simulink model "PubIfDecisionTOS_MDL"  (R2020b)
settings: configuration reference "DspaceConfig" (kept outside this file)
PostLoadFcn:
  | if any(exist('dsrtsu_mdlpostloadfcn', 'file') ~= 0), dsrtsu_mdlpostloadfcn('Execute', bdroot); end
InitFcn:
  | , if any(exist('dsmpb_private', 'file') ~= 0), dsmpb_private('dsmpb_mdlclblib', 'Init', bdroot); end,
undefined symbols (not defined in the file or in its folder): C_TOS_ACCEgoRAxletoFbumplength_m, C_TOS_ACCTargetFront_Flag, C_TOS_AEBJAPedObjDxThre_Val, C_TOS_AEBJAPedObjDyThre_Val, C_TOS_AEBJATargetSize_Val, C_TOS_AEBJAVehObjDxThre_Val, C_TOS_AEBJAVehObjDyThre_Val, C_TOS_AEBJuncPedTargetSize_Val, C_TOS_AEBLatObjDxThre_Val, C_TOS_AEBLatPedDyThre_Val, C_TOS_AEBLatTargetSize_Val, C_TOS_AEBLongTargetInEgoFront_Flag, C_TOS_axAbsGround_Parameter, C_TOS_CameraConfirmedFlag, C_TOS_CNsubjWidth, C_TOS_CurrentLaneCoreMinWidth_Val, C_TOS_CutInProb_Val_Zero, C_TOS_CutOutProb_Val_Zero, C_TOS_D2R_Val, C_TOS_DefaultValueObjectToCenterLine_dy, C_TOS_EgoCarWidth_Val, C_TOS_EgoDxRefPoint_m, C_TOS_EgoRAxletoFbumplength_m, C_TOS_HalfWidthVehicle_Con, C_TOS_HWA_CurrentLaneFlag, C_TOS_HWA_LeftLaneFlag, C_TOS_HWA_MovingDir_Vaild, C_TOS_HWA_MovState_Vaild, C_TOS_HWA_RightLaneFlag, C_TOS_LaneLineCourseErrorFront, C_TOS_LaneLineCourseErrorRear, C_TOS_MotorbikeDefaultWidth_m, C_TOS_NumberOfEffectiveTargets, C_TOS_Obj_Age_Val, C_TOS_Objdx_Constraint_Val, C_TOS_ObjectDefaultWidth_m, C_TOS_ObjInCurrentLane_Val, C_TOS_ObjInCurrentLaneValid, C_TOS_ObjInLeftLaneValid, C_TOS_ObjInRightLaneValid, C_TOS_ObjNotInCurrentLane_Val, C_TOS_ObjNotREElementType, C_TOS_ObjPredictDis_dy_ConstantVal_Zeros, C_TOS_ObjToCenterLine_ConstantVal_Zeros, C_TOS_OFMObjIDInvilad_Val, C_TOS_PIL_LatDisCons_Val_zero, C_TOS_PIL_ObjectCutInFlag_b, C_TOS_PIL_ObjectCutOutFlag_b, C_TOS_PIL_ObjLaneProb_al_Val, C_TOS_PP_ObjFusType_FC_Confirm_b, C_TOS_PP_ObjFusType_FC_FR_Confirm_b, C_TOS_PP_ObjFusType_FR_Confirm_b, C_TOS_RE_80BoolDefault_Val, C_TOS_RE_80Single181Default_Val, C_TOS_RE_80Single255Default_Val, C_TOS_RE_80Uint8Default_Val, C_TOS_RE_D2R, C_TOS_RE_D_180_Val, C_TOS_RE_InvalidObjectID_Val, C_TOS_RE_InvalidTargetChainDir_Val ... (+142)
libraries: simulink x1650, TOS_LIB x361, canfdmsglib x14
(part 19 of 69)

== system PubIfDecisionTOS_MDL/TOS_20201112/TOS_2012080320/TOS/ACC/TOS_ACCCurrentLane/ACC_CurrentLane_Target/TOS_ACC_P1 ==
  ACC_P0_P1_Index : Inport
  Object_ID : Inport  Port=2
  Object_Fus_Type : Inport  Port=3
  object_MovingState : Inport  Port=4
  PP_ObjMovingDirSignalProcessing : Inport  Port=5
  Object_HeadingAngle : Inport  Port=6
  Object_DX : Inport  Port=7
  TOS_TLJ_SameLaneConfirm_Flag : Inport  Port=8
  Object_Type : Inport  Port=9
  Object_ObstacleProb : Inport  Port=10
  Object_DY : Inport  Port=11
  PP_ObjFusType_FC_FR_Confirm : Inport  Port=12
  PP_ObjFusType_FR_Confirm : Inport  Port=13
  PP_ObjFusType_FC_Confirm : Inport  Port=14
  Object_VX : Inport  Port=15
  Object_VY : Inport  Port=16
  VIE_EgoVelocity : Inport  Port=17
  SteerWheelAng : Inport  Port=18
  PIL_OverlapRatio : Inport  Port=19
  ACC_TargetP1_ID_K1 : Inport  Port=20
  ACC_TargetP1_ID_K2 : Inport  Port=21
  ACC_TargetP1_MovState_K1 : Inport  Port=22
  ACC_TargetP1_MovState_K2 : Inport  Port=23
  LM_LR_Line04_dDisStart : Inport  Port=24
  LM_LR_Line04_dDisEnd : Inport  Port=25
  LM_LR_Line05_dDisStart : Inport  Port=26
  LM_LR_Line05_dDisEnd : Inport  Port=27
  LM_LR_Line06_dDisStart : Inport  Port=28
  LM_LR_Line06_dDisEnd : Inport  Port=29
  LM_LR_Line04_pC2 : Inport  Port=30
  LM_LR_Line05_pC2 : Inport  Port=31
  LM_LR_Line06_pC2 : Inport  Port=32
  LM_LR_Line04_fCamValid : Inport  Port=33
  LM_LR_Line05_fCamValid : Inport  Port=34
  LM_LR_Line06_fCamValid : Inport  Port=35
  LM_LR_Line04_pC0 : Inport  Port=36
  LM_RL_Line04_pC0 : Inport  Port=37
  ACC_P1_Targe : Subsystem
  ACC_P1_TargeDefault : Subsystem  TreatAsAtomicUnit=on
  Compare To Constant : simulink/Logic and Bit Operations/Compare To Constant  relop===  const=C_TOS_OFMObjIDInvilad_Val  OutDataTypeStr=boolean
      settings: AttributesFormatString=C_TOS_OFMObjIDInvilad_Val = 0
  Constant1 : Constant  Value=0  OutDataTypeStr=uint8
  If : If  IfExpression=u1 ~= 0
  Merge{,1..18} (19 alike) : Merge
  Selector17 : Selector  InputPortWidth=2  IndexOptions=Index vector (dialog)  Indices=2  OutputSizes=1
  Switch1 : Switch  Criteria=u2 ~= 0
  TOS_ACC_P1_Index : Outport
  TOS_ACC_FusionType_ObserVale : Outport  Port=2
  TOS_ACC_TrgMovDir_ObserVale : Outport  Port=3
  TOS_ACC_TargetDxConfirm_ObserVale : Outport  Port=4
  TOS_ACC_ObjType_ObserVale : Outport  Port=5
  TOS_ACC_ObstacleProb_ObserVale : Outport  Port=6
  TOS_ACC_DyConfirm_ObserVale : Outport  Port=7
  TOS_ACC_TrgMovDirFlag_1_ObserVale : Outport  Port=8
  TOS_ACC_TrgMovDirFlag_2_ObserVale : Outport  Port=9
  TOS_ACC_TrgMovDirFlag_3_ObserVale : Outport  Port=10
  TOS_ACC_TrgMovDirFlag_4_ObserVale : Outport  Port=11
  TOS_ACC_TrgMovDirFlag_5_ObserVale : Outport  Port=12
  TOS_ACC_TrgMovDirFlag_6_ObserVale : Outport  Port=13
  TOS_ACC_DyConfirm_1_ObserVale : Outport  Port=14
  TOS_ACC_DyConfirm_2_ObserVale : Outport  Port=15
  TOS_ACC_DyConfirm_3_ObserVale : Outport  Port=16
  TOS_ACC_DyConfirm_4_OverlapRatio_ObserVale : Outport  Port=17
  TOS_ACC_DyConfirm_5_OverlapConfirm_ObserVale : Outport  Port=18
  TOS_ACC_DyConfirm_ALL_6_ObserVale : Outport  Port=19
  wires:
  LM_RL_Line04_pC0/1 -> ACC_P1_Targe/37(LM_RL_Line04_pC0)  "LM_RL_Line04_pC0"
  LM_LR_Line04_pC0/1 -> ACC_P1_Targe/36(LM_LR_Line04_pC0)  "LM_LR_Line04_pC0"
  ACC_P1_TargeDefault/19(TOS_ACC_DyConfirm_ALL_6_ObserVale1) -> Merge18/1
  Merge18/1 -> TOS_ACC_DyConfirm_ALL_6_ObserVale/1
  ACC_P1_Targe/19(TOS_ACC_DyConfirm_ALL_6_ObserVale) -> Merge18/2
  ACC_P1_TargeDefault/18(TOS_ACC_DyConfirm_5_OverlapConfirm_ObserVale) -> Merge17/1
  ACC_P1_TargeDefault/17(TOS_ACC_DyConfirm_4_OverlapRatio_ObserVale) -> Merge15/1
  ACC_P1_TargeDefault/16(TOS_ACC_DyConfirm_3_ObserVale) -> Merge14/1
  ACC_P1_TargeDefault/15(TOS_ACC_DyConfirm_2_ObserVale) -> Merge13/1
  ACC_P1_TargeDefault/14(TOS_ACC_DyConfirm_1_ObserVale) -> Merge16/1
  ACC_P1_TargeDefault/13(TOS_ACC_TrgMovDirFlag_6_ObserVale) -> Merge8/1
  ACC_P1_TargeDefault/12(TOS_ACC_TrgMovDirFlag_5_ObserVale) -> Merge12/1
  ACC_P1_TargeDefault/11(TOS_ACC_TrgMovDirFlag_4_ObserVale) -> Merge11/1
  ACC_P1_TargeDefault/10(TOS_ACC_TrgMovDirFlag_3_ObserVale) -> Merge10/1
  ACC_P1_TargeDefault/9(TOS_ACC_TrgMovDirFlag_2_ObserVale) -> Merge9/1
  ACC_P1_TargeDefault/8(TOS_ACC_TrgMovDirFlag_1_ObserVale) -> Merge7/1
  ACC_P1_TargeDefault/7(TOS_ACC_DyConfirm_ObserVale) -> Merge6/1
  ACC_P1_TargeDefault/6(TOS_ACC_ObstacleProb_ObserVale) -> Merge5/1
  ACC_P1_TargeDefault/5(TOS_ACC_ObjType_ObserVale) -> Merge4/1
  ACC_P1_TargeDefault/4(TOS_ACC_TargetDxConfirm_ObserVale) -> Merge3/1
  ACC_P1_TargeDefault/3(TOS_ACC_TrgMovDir_ObserVale) -> Merge2/1
  ACC_P1_TargeDefault/2(TOS_ACC_FusionType_ObserVale) -> Merge1/1
  ACC_P1_TargeDefault/1(ACC_P1_TargeConfirm) -> Merge/1
  ACC_P1_Targe/18(TOS_ACC_DyConfirm_5_OverlapConfirm_ObserVale) -> Merge17/2
  Merge17/1 -> TOS_ACC_DyConfirm_5_OverlapConfirm_ObserVale/1
  LM_LR_Line06_fCamValid/1 -> ACC_P1_Targe/35(LM_LR_Line06_fCamValid)
  LM_LR_Line05_fCamValid/1 -> ACC_P1_Targe/34(LM_LR_Line05_fCamValid)
  LM_LR_Line04_fCamValid/1 -> ACC_P1_Targe/33(LM_LR_Line04_fCamValid)
  LM_LR_Line06_pC2/1 -> ACC_P1_Targe/32(LM_LR_Line06_pC2)
  LM_LR_Line05_pC2/1 -> ACC_P1_Targe/31(LM_LR_Line05_pC2)
  LM_LR_Line04_pC2/1 -> ACC_P1_Targe/30(LM_LR_Line04_pC2)
  LM_LR_Line06_dDisEnd/1 -> ACC_P1_Targe/29(LM_LR_Line06_dDisEnd)
  LM_LR_Line06_dDisStart/1 -> ACC_P1_Targe/28(LM_LR_Line06_dDisStart)
  LM_LR_Line05_dDisEnd/1 -> ACC_P1_Targe/27(LM_LR_Line05_dDisEnd)
  LM_LR_Line05_dDisStart/1 -> ACC_P1_Targe/26(LM_LR_Line05_dDisStart)
  LM_LR_Line04_dDisEnd/1 -> ACC_P1_Targe/25(LM_LR_Line04_dDisEnd)
  LM_LR_Line04_dDisStart/1 -> ACC_P1_Targe/24(LM_LR_Line04_dDisStart)
  ACC_P1_Targe/14(TOS_ACC_DyConfirm_1_ObserVale) -> Merge16/2
  Merge16/1 -> TOS_ACC_DyConfirm_1_ObserVale/1
  Switch1/1 -> TOS_ACC_P1_Index/1
  Selector17/1 -> Compare To Constant/1, [ACC_P1_Index]
  Merge15/1 -> TOS_ACC_DyConfirm_4_OverlapRatio_ObserVale/1
  Merge14/1 -> TOS_ACC_DyConfirm_3_ObserVale/1
  Merge13/1 -> TOS_ACC_DyConfirm_2_ObserVale/1
  ACC_P1_Targe/17(TOS_ACC_DyConfirm_4_OverlapRatio_ObserVale) -> Merge15/2
  ACC_P1_Targe/16(TOS_ACC_DyConfirm_3_ObserVale) -> Merge14/2
  ACC_P1_Targe/15(TOS_ACC_DyConfirm_2_ObserVale) -> Merge13/2
  ACC_P1_Targe/12(TOS_ACC_TrgMovDirFlag_5_ObserVale) -> Merge12/2
  ACC_P1_Targe/11(TOS_ACC_TrgMovDirFlag_4_ObserVale) -> Merge11/2
  ACC_P1_Targe/10(TOS_ACC_TrgMovDirFlag_3_ObserVale) -> Merge10/2
  ACC_P1_Targe/9(TOS_ACC_TrgMovDirFlag_2_ObserVale) -> Merge9/2
  Merge12/1 -> TOS_ACC_TrgMovDirFlag_5_ObserVale/1
  Merge11/1 -> TOS_ACC_TrgMovDirFlag_4_ObserVale/1
  Merge10/1 -> TOS_ACC_TrgMovDirFlag_3_ObserVale/1
  Merge9/1 -> TOS_ACC_TrgMovDirFlag_2_ObserVale/1
  Merge8/1 -> TOS_ACC_TrgMovDirFlag_6_ObserVale/1
  ACC_P1_Targe/13(TOS_ACC_TrgMovDirFlag_6_ObserVale) -> Merge8/2
  Object_ID/1 -> ACC_P1_Targe/23(ObjectID)
  ACC_TargetP1_MovState_K2/1 -> ACC_P1_Targe/22(ACC_Target_MovState_K2)
  ACC_TargetP1_MovState_K1/1 -> ACC_P1_Targe/21(ACC_Target_MovState_K1)
  ACC_TargetP1_ID_K2/1 -> ACC_P1_Targe/20(ACC_Target_ID_K2)
  ACC_TargetP1_ID_K1/1 -> ACC_P1_Targe/19(ACC_Target_ID_K1)
  Merge7/1 -> TOS_ACC_TrgMovDirFlag_1_ObserVale/1
  ACC_P1_Targe/8(TOS_ACC_TrgMovDirFlag_1_ObserVale) -> Merge7/2
  PIL_OverlapRatio/1 -> ACC_P1_Targe/18(PIL_OverlapRatio)
  SteerWheelAng/1 -> ACC_P1_Targe/17(SteerWheelAng)
  VIE_EgoVelocity/1 -> ACC_P1_Targe/16(VIE_EgoVelocity)
  Object_VX/1 -> ACC_P1_Targe/14(Object_VX)
  Object_VY/1 -> ACC_P1_Targe/15(Object_VY)
  PP_ObjFusType_FR_Confirm/1 -> ACC_P1_Targe/12(PP_ObjFusType_FR_Confirm)
  PP_ObjFusType_FC_FR_Confirm/1 -> ACC_P1_Targe/11(PP_ObjFusType_FC_FR_Confirm)
  PP_ObjFusType_FC_Confirm/1 -> ACC_P1_Targe/13(PP_ObjFusType_FC_Confirm)
  If/2 -> ACC_P1_Targe/Action
  ACC_P1_Targe/7(TOS_ACC_DyConfirm_ObserVale) -> Merge6/2
  ACC_P1_Targe/6(TOS_ACC_ObstacleProb_ObserVale) -> Merge5/2
  ACC_P1_Targe/5(TOS_ACC_ObjType_ObserVale) -> Merge4/2
  ACC_P1_Targe/4(TOS_ACC_TargetDxConfirm_ObserVale) -> Merge3/2
  ACC_P1_Targe/3(TOS_ACC_TrgMovDir_ObserVale) -> Merge2/2
  ACC_P1_Targe/2(TOS_ACC_FusionType_ObserVale) -> Merge1/2
  ACC_P1_Targe/1(ACC_P1_TargeConfirm) -> Merge/2
  Object_DY/1 -> ACC_P1_Targe/10(Object_DY)
  Object_ObstacleProb/1 -> ACC_P1_Targe/9(Object_ObstacleProb)
  Object_Type/1 -> ACC_P1_Targe/8(Object_Type)
  TOS_TLJ_SameLaneConfirm_Flag/1 -> ACC_P1_Targe/7(TOS_TLJ_SameLaneConfirm_Flag)
  Object_DX/1 -> ACC_P1_Targe/6(Object_DX)
  Object_HeadingAngle/1 -> ACC_P1_Targe/5(Object_HeadingAngle)
  PP_ObjMovingDirSignalProcessing/1 -> ACC_P1_Targe/4(PP_ObjMovingDirSignalProcessing)
  object_MovingState/1 -> ACC_P1_Targe/3(object_MovingState)
  Object_Fus_Type/1 -> ACC_P1_Targe/2(Object_Fus_Type)
  [ACC_P1_Index] -> ACC_P1_Targe/1(ACC_P1_Index)
  ACC_P0_P1_Index/1 -> Selector17/1
  Constant1/1 -> Switch1/3
  Merge/1 -> Switch1/2
  [ACC_P1_Index] -> Switch1/1
  Merge6/1 -> TOS_ACC_DyConfirm_ObserVale/1
  Merge5/1 -> TOS_ACC_ObstacleProb_ObserVale/1
  Merge4/1 -> TOS_ACC_ObjType_ObserVale/1
  Merge3/1 -> TOS_ACC_TargetDxConfirm_ObserVale/1
  Merge2/1 -> TOS_ACC_TrgMovDir_ObserVale/1
  Merge1/1 -> TOS_ACC_FusionType_ObserVale/1
  Compare To Constant/1 -> If/1
  If/1 -> ACC_P1_TargeDefault/Action

== system PubIfDecisionTOS_MDL/TOS_20201112/TOS_2012080320/TOS/ACC/TOS_ACCCurrentLane/ACC_Object_PreConfirm/ACC_P0_P1_Object_TargPreConfirm ==
  PP_ObjFusType_FC_FR_Confirm : Inport  Partition=on  PartitionDimension=1  PartitionWidth=1  PartitionOffset=0
  PP_ObjFusType_FR_Confirm : Inport  Port=2  Partition=on  PartitionDimension=1  PartitionWidth=1  PartitionOffset=0
  PP_ObjFusType_FC_Confirm : Inport  Port=3  Partition=on  PartitionDimension=1  PartitionWidth=1  PartitionOffset=0
  Object_ID : Inport  Port=4  OutDataTypeStr=uint8  Partition=on  PartitionDimension=1  PartitionWidth=1  PartitionOffset=0
  Obj_MovingState : Inport  Port=5  Partition=on  PartitionDimension=1  PartitionWidth=1  PartitionOffset=0
  Obj_Dx : Inport  Port=6  Partition=on  PartitionDimension=1  PartitionWidth=1  PartitionOffset=0
  Object_ObstacleProb : Inport  Port=7  Partition=on  PartitionDimension=1  PartitionWidth=1  PartitionOffset=0
  Object_DY : Inport  Port=8  Partition=on  PartitionDimension=1  PartitionWidth=1  PartitionOffset=0
  Object_ObjType : Inport  Port=9  Partition=on  PartitionDimension=1  PartitionWidth=1  PartitionOffset=0
  TOS_TLJ_SameLaneConfirm_Flag : Inport  Port=10  Partition=on  PartitionDimension=1  PartitionWidth=1  PartitionOffset=0
  LM_LR_Line04_fCamValid : Inport  Port=11
  LM_LR_Line05_fCamValid : Inport  Port=12
  LM_LR_Line06_fCamValid : Inport  Port=13
  ACC_TargetP0_ID_K1 : Inport  Port=14
  ACC_TargetP0_Dx_K1 : Inport  Port=15
  PIL_OverlapRatio : Inport  Port=16  Partition=on  PartitionDimension=1  PartitionWidth=1  PartitionOffset=0
  PIL_OverlapRatio_K1 : Inport  Port=17  Partition=on  PartitionDimension=1  PartitionWidth=1  PartitionOffset=0
  PIL_OverlapRatio_K2 : Inport  Port=18  Partition=on  PartitionDimension=1  PartitionWidth=1  PartitionOffset=0
  LM_LR_Line04_dDisStart : Inport  Port=19
  LM_LR_Line04_dDisEnd : Inport  Port=20
  LM_LR_Line05_dDisStart : Inport  Port=21
  LM_LR_Line05_dDisEnd : Inport  Port=22
  LM_LR_Line06_dDisStart : Inport  Port=23
  LM_LR_Line06_dDisEnd : Inport  Port=24
  PP_REElementType : Inport  Port=25  Partition=on  PartitionDimension=1  PartitionWidth=1  PartitionOffset=0
  ACC_P0_P1_Object_TargPreConfirm : Subsystem
  ACC_P0_P1_Object_TargPreConfirmDefault : Subsystem  TreatAsAtomicUnit=on
  Compare To Constant : simulink/Logic and Bit Operations/Compare To Constant  relop===  const=C_TOS_OFMObjIDInvilad_Val  OutDataTypeStr=boolean
      settings: AttributesFormatString=C_TOS_OFMObjIDInvilad_Val = 0
  For Each : ForEach  DisableCoverage=on
  If : If  IfExpression=u1 ~= 0
  Merge{,1..10} (11 alike) : Merge
  TOS_ACC_P0_P1_TargetPre_1_ConditionFlag_ObserVale : Outport  ConcatenationDimension=1
  TOS_ACC_P0_P1_TargetPre_2_OverlapThre_ObserVale : Outport  Port=2  ConcatenationDimension=1
  TOS_ACC_P0_P1_TargetPre_3_SameLane_Flag_ObserVale : Outport  Port=3  ConcatenationDimension=1
  TOS_ACC_P0_P1_TargetPre_SameLaneFlag : Outport  Port=4  ConcatenationDimension=1
  TOS_ACC_P0_P1_TargetPre_FiltFlag : Outport  Port=5  ConcatenationDimension=1
  TOS_ACC_P0_P1_TargetPre_FusionTypeFlag_ObserVale : Outport  Port=6  ConcatenationDimension=1
  TOS_ACC_P0_P1_TargetPre_PassedbyTarget_Flag_ObserVale : Outport  Port=7  ConcatenationDimension=1
  TOS_ACC_P0_P1_TargetPre_FenceFlag_ObserVale : Outport  Port=8  ConcatenationDimension=1
  TOS_ACC_P0_P1_TargetPre_ObjType_ObserVale : Outport  Port=9  ConcatenationDimension=1
  TOS_ACC_P0_P1_TargetPre_OverlapThre_Val_ObserVale : Outport  Port=10  ConcatenationDimension=1
  TOS_ACC_P0_P1_TargetPre_REElementType_ObserVale : Outport  Port=11  ConcatenationDimension=1
  wires:
  PP_ObjFusType_FC_FR_Confirm/1 -> ACC_P0_P1_Object_TargPreConfirm/2(PP_ObjFusType_FC_FR_Confirm)
  PP_ObjFusType_FR_Confirm/1 -> ACC_P0_P1_Object_TargPreConfirm/3(PP_ObjFusType_FR_Confirm)
  Compare To Constant/1 -> If/1
  Object_ID/1 -> [Object_ID], Compare To Constant/1
  If/1 -> ACC_P0_P1_Object_TargPreConfirmDefault/Action
  If/2 -> ACC_P0_P1_Object_TargPreConfirm/Action
  PP_ObjFusType_FC_Confirm/1 -> ACC_P0_P1_Object_TargPreConfirm/4(PP_ObjFusType_FC_Confirm)
  Obj_MovingState/1 -> ACC_P0_P1_Object_TargPreConfirm/5(Obj_MovingState)
  Obj_Dx/1 -> ACC_P0_P1_Object_TargPreConfirm/6(Obj_Dx)
  Object_ObstacleProb/1 -> ACC_P0_P1_Object_TargPreConfirm/7(Object_ObstacleProb)
  Object_DY/1 -> ACC_P0_P1_Object_TargPreConfirm/8(Object_DY)
  ACC_TargetP0_ID_K1/1 -> ACC_P0_P1_Object_TargPreConfirm/14(ACC_TargetP0_ID_K1)
  ACC_TargetP0_Dx_K1/1 -> ACC_P0_P1_Object_TargPreConfirm/15(ACC_TargetP0_Dx_K1)
  [Object_ID] -> ACC_P0_P1_Object_TargPreConfirm/1(Object_ID)
  Object_ObjType/1 -> ACC_P0_P1_Object_TargPreConfirm/9(Object_ObjType)
  PIL_OverlapRatio/1 -> ACC_P0_P1_Object_TargPreConfirm/16(PIL_OverlapRatio)
  TOS_TLJ_SameLaneConfirm_Flag/1 -> ACC_P0_P1_Object_TargPreConfirm/10(TOS_TLJ_SameLaneConfirm_Flag)
  Merge/1 -> TOS_ACC_P0_P1_TargetPre_1_ConditionFlag_ObserVale/1
  Merge1/1 -> TOS_ACC_P0_P1_TargetPre_2_OverlapThre_ObserVale/1
  Merge2/1 -> TOS_ACC_P0_P1_TargetPre_3_SameLane_Flag_ObserVale/1
  Merge3/1 -> TOS_ACC_P0_P1_TargetPre_SameLaneFlag/1
  Merge4/1 -> TOS_ACC_P0_P1_TargetPre_FiltFlag/1
  Merge5/1 -> TOS_ACC_P0_P1_TargetPre_FusionTypeFlag_ObserVale/1
  Merge6/1 -> TOS_ACC_P0_P1_TargetPre_PassedbyTarget_Flag_ObserVale/1
  Merge7/1 -> TOS_ACC_P0_P1_TargetPre_ObjType_ObserVale/1
  Merge8/1 -> TOS_ACC_P0_P1_TargetPre_OverlapThre_Val_ObserVale/1
  ACC_P0_P1_Object_TargPreConfirm/1(TOS_ACC_P0_P1_TargetPre_1_ConditionFlag_ObserVale) -> Merge/2
  ACC_P0_P1_Object_TargPreConfirm/10(TOS_ACC_P0_P1_TargetPre_OverlapThre_Val_ObserVale) -> Merge8/2
  ACC_P0_P1_Object_TargPreConfirm/2(TOS_ACC_P0_P1_TargetPre_2_OverlapThre_ObserVale) -> Merge1/2
  ACC_P0_P1_Object_TargPreConfirm/3(TOS_ACC_P0_P1_TargetPre_3_SameLane_Flag_ObserVale) -> Merge2/2
  ACC_P0_P1_Object_TargPreConfirm/4(TOS_ACC_P0_P1_TargetPre_SameLaneFlag) -> Merge3/2
  ACC_P0_P1_Object_TargPreConfirm/5(TOS_ACC_P0_P1_TargetPre_FiltFlag) -> Merge4/2
  ACC_P0_P1_Object_TargPreConfirm/6(TOS_ACC_P0_P1_TargetPre_FusionTypeFlag_ObserVale) -> Merge5/2
  ACC_P0_P1_Object_TargPreConfirm/7(TOS_ACC_P0_P1_TargetPre_PassedbyTarget_Flag_ObserVale) -> Merge6/2
  ACC_P0_P1_Object_TargPreConfirm/8(TOS_ACC_P0_P1_TargetPre_FenceFlag_ObserVale) -> Merge9/2
  ACC_P0_P1_Object_TargPreConfirm/9(TOS_ACC_P0_P1_TargetPre_ObjType_ObserVale) -> Merge7/2
  ACC_P0_P1_Object_TargPreConfirmDefault/1(TOS_ACC_P0_P1_TargetPre_1_ConditionFlag_ObserVale) -> Merge/1
  ACC_P0_P1_Object_TargPreConfirmDefault/2(TOS_ACC_P0_P1_TargetPre_2_OverlapThre_ObserVale) -> Merge1/1
  ACC_P0_P1_Object_TargPreConfirmDefault/3(TOS_ACC_P0_P1_TargetPre_3_SameLane_Flag_ObserVale) -> Merge2/1
  ACC_P0_P1_Object_TargPreConfirmDefault/4(TOS_ACC_P0_P1_TargetPre_SameLaneFlag) -> Merge3/1
  ACC_P0_P1_Object_TargPreConfirmDefault/5(TOS_ACC_P0_P1_TargetPre_FiltFlag) -> Merge4/1
  ACC_P0_P1_Object_TargPreConfirmDefault/6(TOS_ACC_P0_P1_TargetPre_FusionTypeFlag_ObserVale) -> Merge5/1
  ACC_P0_P1_Object_TargPreConfirmDefault/7(TOS_ACC_P0_P1_TargetPre_PassedbyTarget_Flag_ObserVale) -> Merge6/1
  ACC_P0_P1_Object_TargPreConfirmDefault/8(TOS_ACC_P0_P1_TargetPre_FenceFlag_ObserVale) -> Merge9/1
  ACC_P0_P1_Object_TargPreConfirmDefault/9(TOS_ACC_P0_P1_TargetPre_ObjType_ObserVale) -> Merge7/1
  ACC_P0_P1_Object_TargPreConfirmDefault/10(TOS_ACC_P0_P1_TargetPre_OverlapThre_Val_ObserVale) -> Merge8/1
  Merge9/1 -> TOS_ACC_P0_P1_TargetPre_FenceFlag_ObserVale/1
  PIL_OverlapRatio_K1/1 -> ACC_P0_P1_Object_TargPreConfirm/17(PIL_OverlapRatio_K1)
  PIL_OverlapRatio_K2/1 -> ACC_P0_P1_Object_TargPreConfirm/18(PIL_OverlapRatio_K2)
  LM_LR_Line04_fCamValid/1 -> ACC_P0_P1_Object_TargPreConfirm/11(LM_LR_Line04_fCamValid)
  LM_LR_Line05_fCamValid/1 -> ACC_P0_P1_Object_TargPreConfirm/12(LM_LR_Line05_fCamValid)
  LM_LR_Line06_fCamValid/1 -> ACC_P0_P1_Object_TargPreConfirm/13(LM_LR_Line06_fCamValid)
  LM_LR_Line04_dDisStart/1 -> ACC_P0_P1_Object_TargPreConfirm/19(LM_LR_Line04_dDisStart)
  LM_LR_Line04_dDisEnd/1 -> ACC_P0_P1_Object_TargPreConfirm/20(LM_LR_Line04_dDisEnd)
  LM_LR_Line05_dDisStart/1 -> ACC_P0_P1_Object_TargPreConfirm/21(LM_LR_Line05_dDisStart)
  LM_LR_Line05_dDisEnd/1 -> ACC_P0_P1_Object_TargPreConfirm/22(LM_LR_Line05_dDisEnd)
  LM_LR_Line06_dDisStart/1 -> ACC_P0_P1_Object_TargPreConfirm/23(LM_LR_Line06_dDisStart)
  LM_LR_Line06_dDisEnd/1 -> ACC_P0_P1_Object_TargPreConfirm/24(LM_LR_Line06_dDisEnd)
  PP_REElementType/1 -> ACC_P0_P1_Object_TargPreConfirm/25(PP_REElementType)
  Merge10/1 -> TOS_ACC_P0_P1_TargetPre_REElementType_ObserVale/1
  ACC_P0_P1_Object_TargPreConfirm/11(TOS_ACC_P0_P1_TargetPre_REElementType_ObserVale) -> Merge10/2
  ACC_P0_P1_Object_TargPreConfirmDefault/11(TOS_ACC_P0_P1_TargetPre_REElementType_ObserVale) -> Merge10/1

== system PubIfDecisionTOS_MDL/TOS_20201112/TOS_2012080320/TOS/ACC/TOS_ACCLeftLane/ACC_LeftLane_Target/TOS_ACC_P2 ==
  TOS_ACC_P2_P4_Index : Inport
  Object_ID : Inport  Port=2
  Object_Fus_Type : Inport  Port=3
  object_MovingState : Inport  Port=4
  PP_ObjMovingDirSignalProcessing : Inport  Port=5
  Object_HeadingAngle : Inport  Port=6
  Object_DX : Inport  Port=7
  Object_Type : Inport  Port=8
  Object_ObstacleProb : Inport  Port=9
  Object_DY : Inport  Port=10
  PP_ObjFusType_FC_FR_Confirm : Inport  Port=11
  PP_ObjFusType_FR_Confirm : Inport  Port=12
  PP_ObjFusType_FC_Confirm : Inport  Port=13
  Object_VX : Inport  Port=14
  Object_VY : Inport  Port=15
  VIE_EgoVelocity : Inport  Port=16
  SteerWheelAng : Inport  Port=17
  ACC_TargetP2_ID_K1 : Inport  Port=18
  ACC_TargetP2_ID_K2 : Inport  Port=19
  ACC_TargetP2_MovState_K1 : Inport  Port=20
  ACC_TargetP2_MovState_K2 : Inport  Port=21
  ACC_P2_Targe : Subsystem
  ACC_P2_TargeDefault : Subsystem  TreatAsAtomicUnit=on
  Compare To Constant : simulink/Logic and Bit Operations/Compare To Constant  relop===  const=C_TOS_OFMObjIDInvilad_Val  OutDataTypeStr=boolean
      settings: AttributesFormatString=C_TOS_OFMObjIDInvilad_Val = 0
  Constant1 : Constant  Value=0  OutDataTypeStr=uint8
  If : If  IfExpression=u1 ~= 0
  Merge{,1..5,7..12} (12 alike) : Merge
  Selector17 : Selector  InputPortWidth=2  IndexOptions=Index vector (dialog)  Indices=1  OutputSizes=1
  Switch1 : Switch  Criteria=u2 ~= 0
  TOS_ACC_P2_Index : Outport
  TOS_ACC_FusionType_ObserVale : Outport  Port=2
  TOS_ACC_TrgMovDir_ObserVale : Outport  Port=3
  TOS_ACC_TargetDxConfirm_ObserVale : Outport  Port=4
  TOS_ACC_ObjType_ObserVale : Outport  Port=5
  TOS_ACC_ObstacleProb_ObserVale : Outport  Port=6
  TOS_ACC_TrgMovDirFlag_1_ObserVale : Outport  Port=7
  TOS_ACC_TrgMovDirFlag_2_ObserVale : Outport  Port=8
  TOS_ACC_TrgMovDirFlag_3_ObserVale : Outport  Port=9
  TOS_ACC_TrgMovDirFlag_4_ObserVale : Outport  Port=10
  TOS_ACC_TrgMovDirFlag_5_ObserVale : Outport  Port=11
  TOS_ACC_TrgMovDirFlag_6_ObserVale : Outport  Port=12
  wires:
  ACC_P2_TargeDefault/12(TOS_ACC_TrgMovDirFlag_6_ObserVale) -> Merge8/1
  ACC_P2_TargeDefault/11(TOS_ACC_TrgMovDirFlag_5_ObserVale) -> Merge12/1
  ACC_P2_TargeDefault/10(TOS_ACC_TrgMovDirFlag_4_ObserVale) -> Merge11/1
  ACC_P2_TargeDefault/9(TOS_ACC_TrgMovDirFlag_3_ObserVale) -> Merge10/1
  ACC_P2_TargeDefault/8(TOS_ACC_TrgMovDirFlag_2_ObserVale) -> Merge9/1
  ACC_P2_TargeDefault/7(TOS_ACC_TrgMovDirFlag_1_ObserVale) -> Merge7/1
  ACC_P2_TargeDefault/6(TOS_ACC_ObstacleProb_ObserVale) -> Merge5/1
  ACC_P2_TargeDefault/5(TOS_ACC_ObjType_ObserVale) -> Merge4/1
  ACC_P2_TargeDefault/4(TOS_ACC_TargetDxConfirm_ObserVale) -> Merge3/1
  ACC_P2_TargeDefault/3(TOS_ACC_TrgMovDir_ObserVale) -> Merge2/1
  ACC_P2_TargeDefault/2(TOS_ACC_FusionType_ObserVale) -> Merge1/1
  ACC_P2_TargeDefault/1(ACC_P2_TargeConfirm) -> Merge/1
  Switch1/1 -> TOS_ACC_P2_Index/1
  Selector17/1 -> Compare To Constant/1, [ACC_P2_Index]
  ACC_P2_Targe/11(TOS_ACC_TrgMovDirFlag_5_ObserVale) -> Merge12/2
  ACC_P2_Targe/10(TOS_ACC_TrgMovDirFlag_4_ObserVale) -> Merge11/2
  ACC_P2_Targe/9(TOS_ACC_TrgMovDirFlag_3_ObserVale) -> Merge10/2
  ACC_P2_Targe/8(TOS_ACC_TrgMovDirFlag_2_ObserVale) -> Merge9/2
  Merge12/1 -> TOS_ACC_TrgMovDirFlag_5_ObserVale/1
  Merge11/1 -> TOS_ACC_TrgMovDirFlag_4_ObserVale/1
  Merge10/1 -> TOS_ACC_TrgMovDirFlag_3_ObserVale/1
  Merge9/1 -> TOS_ACC_TrgMovDirFlag_2_ObserVale/1
  Merge8/1 -> TOS_ACC_TrgMovDirFlag_6_ObserVale/1
  ACC_P2_Targe/12(TOS_ACC_TrgMovDirFlag_6_ObserVale) -> Merge8/2
  Object_ID/1 -> ACC_P2_Targe/21(ObjectID)
  ACC_TargetP2_MovState_K2/1 -> ACC_P2_Targe/20(ACC_Target_MovState_K2)
  ACC_TargetP2_MovState_K1/1 -> ACC_P2_Targe/19(ACC_Target_MovState_K1)
  ACC_TargetP2_ID_K2/1 -> ACC_P2_Targe/18(ACC_Target_ID_K2)
  ACC_TargetP2_ID_K1/1 -> ACC_P2_Targe/17(ACC_Target_ID_K1)
  Merge7/1 -> TOS_ACC_TrgMovDirFlag_1_ObserVale/1
  ACC_P2_Targe/7(TOS_ACC_TrgMovDirFlag_1_ObserVale) -> Merge7/2
  SteerWheelAng/1 -> ACC_P2_Targe/16(SteerWheelAng)
  VIE_EgoVelocity/1 -> ACC_P2_Targe/15(VIE_EgoVelocity)
  Object_VX/1 -> ACC_P2_Targe/13(Object_VX)
  Object_VY/1 -> ACC_P2_Targe/14(Object_VY)
  PP_ObjFusType_FR_Confirm/1 -> ACC_P2_Targe/11(PP_ObjFusType_FR_Confirm)
  PP_ObjFusType_FC_FR_Confirm/1 -> ACC_P2_Targe/10(PP_ObjFusType_FC_FR_Confirm)
  PP_ObjFusType_FC_Confirm/1 -> ACC_P2_Targe/12(PP_ObjFusType_FC_Confirm)
  If/2 -> ACC_P2_Targe/Action
  ACC_P2_Targe/6(TOS_ACC_ObstacleProb_ObserVale) -> Merge5/2
  ACC_P2_Targe/5(TOS_ACC_ObjType_ObserVale) -> Merge4/2
  ACC_P2_Targe/4(TOS_ACC_TargetDxConfirm_ObserVale) -> Merge3/2
  ACC_P2_Targe/3(TOS_ACC_TrgMovDir_ObserVale) -> Merge2/2
  ACC_P2_Targe/2(TOS_ACC_FusionType_ObserVale) -> Merge1/2
  ACC_P2_Targe/1(ACC_P2_TargeConfirm) -> Merge/2
  Object_DY/1 -> ACC_P2_Targe/9(Object_DY)
  Object_ObstacleProb/1 -> ACC_P2_Targe/8(Object_ObstacleProb)
  Object_Type/1 -> ACC_P2_Targe/7(Object_Type)
  Object_DX/1 -> ACC_P2_Targe/6(Object_DX)
  Object_HeadingAngle/1 -> ACC_P2_Targe/5(Object_HeadingAngle)
  PP_ObjMovingDirSignalProcessing/1 -> ACC_P2_Targe/4(PP_ObjMovingDirSignalProcessing)
  object_MovingState/1 -> ACC_P2_Targe/3(object_MovingState)
  Object_Fus_Type/1 -> ACC_P2_Targe/2(Object_Fus_Type)
  [ACC_P2_Index] -> ACC_P2_Targe/1(ACC_P2_Index)
  TOS_ACC_P2_P4_Index/1 -> Selector17/1
  Constant1/1 -> Switch1/3
  Merge/1 -> Switch1/2
  [ACC_P2_Index] -> Switch1/1
  Merge5/1 -> TOS_ACC_ObstacleProb_ObserVale/1
  Merge4/1 -> TOS_ACC_ObjType_ObserVale/1
  Merge3/1 -> TOS_ACC_TargetDxConfirm_ObserVale/1
  Merge2/1 -> TOS_ACC_TrgMovDir_ObserVale/1
  Merge1/1 -> TOS_ACC_FusionType_ObserVale/1
  Compare To Constant/1 -> If/1
  If/1 -> ACC_P2_TargeDefault/Action

== system PubIfDecisionTOS_MDL/TOS_20201112/TOS_2012080320/TOS/ACC/TOS_ACCLeftLane/ACC_LeftLane_Target/TOS_ACC_P4 ==
  TOS_ACC_P2_P4_Index : Inport
  Object_ID : Inport  Port=2
  Object_Fus_Type : Inport  Port=3
  object_MovingState : Inport  Port=4
  PP_ObjMovingDirSignalProcessing : Inport  Port=5
  Object_HeadingAngle : Inport  Port=6
  Object_DX : Inport  Port=7
  Object_Type : Inport  Port=8
  Object_ObstacleProb : Inport  Port=9
  Object_DY : Inport  Port=10
  PP_ObjFusType_FC_FR_Confirm : Inport  Port=11
  PP_ObjFusType_FR_Confirm : Inport  Port=12
  PP_ObjFusType_FC_Confirm : Inport  Port=13
  Object_VX : Inport  Port=14
  Object_VY : Inport  Port=15
  VIE_EgoVelocity : Inport  Port=16
  SteerWheelAng : Inport  Port=17
  ACC_TargetP4_ID_K1 : Inport  Port=18
  ACC_TargetP4_ID_K2 : Inport  Port=19
  ACC_TargetP4_MovState_K1 : Inport  Port=20
  ACC_TargetP4_MovState_K2 : Inport  Port=21
  ACC_P4_Targe : Subsystem
  ACC_P4_TargeDefault : Subsystem  TreatAsAtomicUnit=on
  Compare To Constant : simulink/Logic and Bit Operations/Compare To Constant  relop===  const=C_TOS_OFMObjIDInvilad_Val  OutDataTypeStr=boolean
      settings: AttributesFormatString=C_TOS_OFMObjIDInvilad_Val = 0
  Constant1 : Constant  Value=0  OutDataTypeStr=uint8
  If : If  IfExpression=u1 ~= 0
  Merge{,1..5,7..12} (12 alike) : Merge
  Selector17 : Selector  InputPortWidth=2  IndexOptions=Index vector (dialog)  Indices=2  OutputSizes=1
  Switch1 : Switch  Criteria=u2 ~= 0
  TOS_ACC_P4_Index : Outport
  TOS_ACC_FusionType_ObserVale : Outport  Port=2
  TOS_ACC_TrgMovDir_ObserVale : Outport  Port=3
  TOS_ACC_TargetDxConfirm_ObserVale : Outport  Port=4
  TOS_ACC_ObjType_ObserVale : Outport  Port=5
  TOS_ACC_ObstacleProb_ObserVale : Outport  Port=6
  TOS_ACC_TrgMovDirFlag_1_ObserVale : Outport  Port=7
  TOS_ACC_TrgMovDirFlag_2_ObserVale : Outport  Port=8
  TOS_ACC_TrgMovDirFlag_3_ObserVale : Outport  Port=9
  TOS_ACC_TrgMovDirFlag_4_ObserVale : Outport  Port=10
  TOS_ACC_TrgMovDirFlag_5_ObserVale : Outport  Port=11
  TOS_ACC_TrgMovDirFlag_6_ObserVale : Outport  Port=12
  wires:
  If/1 -> ACC_P4_TargeDefault/Action
  Compare To Constant/1 -> If/1
  Merge1/1 -> TOS_ACC_FusionType_ObserVale/1
  Merge2/1 -> TOS_ACC_TrgMovDir_ObserVale/1
  Merge3/1 -> TOS_ACC_TargetDxConfirm_ObserVale/1
  Merge4/1 -> TOS_ACC_ObjType_ObserVale/1
  Merge5/1 -> TOS_ACC_ObstacleProb_ObserVale/1
  [ACC_P4_Index] -> Switch1/1
  Merge/1 -> Switch1/2
  Constant1/1 -> Switch1/3
  TOS_ACC_P2_P4_Index/1 -> Selector17/1
  [ACC_P4_Index] -> ACC_P4_Targe/1(ACC_P4_Index)
  Object_Fus_Type/1 -> ACC_P4_Targe/2(Object_Fus_Type)
  object_MovingState/1 -> ACC_P4_Targe/3(object_MovingState)
  PP_ObjMovingDirSignalProcessing/1 -> ACC_P4_Targe/4(PP_ObjMovingDirSignalProcessing)
  Object_HeadingAngle/1 -> ACC_P4_Targe/5(Object_HeadingAngle)
  Object_DX/1 -> ACC_P4_Targe/6(Object_DX)
  Object_Type/1 -> ACC_P4_Targe/7(Object_Type)
  Object_ObstacleProb/1 -> ACC_P4_Targe/8(Object_ObstacleProb)
  Object_DY/1 -> ACC_P4_Targe/9(Object_DY)
  ACC_P4_Targe/1(ACC_P4_TargeConfirm) -> Merge/2
  ACC_P4_Targe/2(TOS_ACC_FusionType_ObserVale) -> Merge1/2
  ACC_P4_Targe/3(TOS_ACC_TrgMovDir_ObserVale) -> Merge2/2
  ACC_P4_Targe/4(TOS_ACC_TargetDxConfirm_ObserVale) -> Merge3/2
  ACC_P4_Targe/5(TOS_ACC_ObjType_ObserVale) -> Merge4/2
  ACC_P4_Targe/6(TOS_ACC_ObstacleProb_ObserVale) -> Merge5/2
  If/2 -> ACC_P4_Targe/Action
  PP_ObjFusType_FC_Confirm/1 -> ACC_P4_Targe/12(PP_ObjFusType_FC_Confirm)
  PP_ObjFusType_FC_FR_Confirm/1 -> ACC_P4_Targe/10(PP_ObjFusType_FC_FR_Confirm)
  PP_ObjFusType_FR_Confirm/1 -> ACC_P4_Targe/11(PP_ObjFusType_FR_Confirm)
  Object_VY/1 -> ACC_P4_Targe/14(Object_VY)
  Object_VX/1 -> ACC_P4_Targe/13(Object_VX)
  VIE_EgoVelocity/1 -> ACC_P4_Targe/15(VIE_EgoVelocity)
  SteerWheelAng/1 -> ACC_P4_Targe/16(SteerWheelAng)
  ACC_P4_Targe/7(TOS_ACC_TrgMovDirFlag_1_ObserVale) -> Merge7/2
  Merge7/1 -> TOS_ACC_TrgMovDirFlag_1_ObserVale/1
  ACC_TargetP4_ID_K1/1 -> ACC_P4_Targe/17(ACC_Target_ID_K1)
  ACC_TargetP4_ID_K2/1 -> ACC_P4_Targe/18(ACC_Target_ID_K2)
  ACC_TargetP4_MovState_K1/1 -> ACC_P4_Targe/19(ACC_Target_MovState_K1)
  ACC_TargetP4_MovState_K2/1 -> ACC_P4_Targe/20(ACC_Target_MovState_K2)
  Object_ID/1 -> ACC_P4_Targe/21(ObjectID)
  ACC_P4_Targe/12(TOS_ACC_TrgMovDirFlag_6_ObserVale) -> Merge8/2
  Merge8/1 -> TOS_ACC_TrgMovDirFlag_6_ObserVale/1
  Merge9/1 -> TOS_ACC_TrgMovDirFlag_2_ObserVale/1
  Merge10/1 -> TOS_ACC_TrgMovDirFlag_3_ObserVale/1
  Merge11/1 -> TOS_ACC_TrgMovDirFlag_4_ObserVale/1
  Merge12/1 -> TOS_ACC_TrgMovDirFlag_5_ObserVale/1
  ACC_P4_Targe/8(TOS_ACC_TrgMovDirFlag_2_ObserVale) -> Merge9/2
  ACC_P4_Targe/9(TOS_ACC_TrgMovDirFlag_3_ObserVale) -> Merge10/2
  ACC_P4_Targe/10(TOS_ACC_TrgMovDirFlag_4_ObserVale) -> Merge11/2
  ACC_P4_Targe/11(TOS_ACC_TrgMovDirFlag_5_ObserVale) -> Merge12/2
  Selector17/1 -> [ACC_P4_Index], Compare To Constant/1
  Switch1/1 -> TOS_ACC_P4_Index/1
  ACC_P4_TargeDefault/1(ACC_P4_TargeConfirm) -> Merge/1
  ACC_P4_TargeDefault/2(TOS_ACC_FusionType_ObserVale) -> Merge1/1
  ACC_P4_TargeDefault/3(TOS_ACC_TrgMovDir_ObserVale) -> Merge2/1
  ACC_P4_TargeDefault/4(TOS_ACC_TargetDxConfirm_ObserVale) -> Merge3/1
  ACC_P4_TargeDefault/5(TOS_ACC_ObjType_ObserVale) -> Merge4/1
  ACC_P4_TargeDefault/6(TOS_ACC_ObstacleProb_ObserVale) -> Merge5/1
  ACC_P4_TargeDefault/7(TOS_ACC_TrgMovDirFlag_1_ObserVale) -> Merge7/1
  ACC_P4_TargeDefault/8(TOS_ACC_TrgMovDirFlag_2_ObserVale) -> Merge9/1
  ACC_P4_TargeDefault/9(TOS_ACC_TrgMovDirFlag_3_ObserVale) -> Merge10/1
  ACC_P4_TargeDefault/10(TOS_ACC_TrgMovDirFlag_4_ObserVale) -> Merge11/1
  ACC_P4_TargeDefault/11(TOS_ACC_TrgMovDirFlag_5_ObserVale) -> Merge12/1
  ACC_P4_TargeDefault/12(TOS_ACC_TrgMovDirFlag_6_ObserVale) -> Merge8/1

== system PubIfDecisionTOS_MDL/TOS_20201112/TOS_2012080320/TOS/ACC/TOS_ACCLeftLane/ACC_Object_PreConfirm/ACC_Object_PreConfirm ==
  PP_ObjFusType_FC_FR_Confirm : Inport  Partition=on  PartitionDimension=1  PartitionWidth=1  PartitionOffset=0
  PP_ObjFusType_FR_Confirm : Inport  Port=2  Partition=on  PartitionDimension=1  PartitionWidth=1  PartitionOffset=0
  PP_ObjFusType_FC_Confirm : Inport  Port=3  Partition=on  PartitionDimension=1  PartitionWidth=1  PartitionOffset=0
  Object_ID : Inport  Port=4  OutDataTypeStr=uint8  Partition=on  PartitionDimension=1  PartitionWidth=1  PartitionOffset=0
  Obj_MovingState : Inport  Port=5  Partition=on  PartitionDimension=1  PartitionWidth=1  PartitionOffset=0
  Obj_Dx : Inport  Port=6  Partition=on  PartitionDimension=1  PartitionWidth=1  PartitionOffset=0
  Object_ObstacleProb : Inport  Port=7  Partition=on  PartitionDimension=1  PartitionWidth=1  PartitionOffset=0
  Object_DY : Inport  Port=8  Partition=on  PartitionDimension=1  PartitionWidth=1  PartitionOffset=0
  Object_ObjType : Inport  Port=9  Partition=on  PartitionDimension=1  PartitionWidth=1  PartitionOffset=0
  ACC_Target_ID_K1 : Inport  Port=10
  ACC_Target_Dx_K1 : Inport  Port=11
  ACC_Object_PreConfirm : Subsystem
  ACC_Object_PreConfirmDefault : Subsystem  TreatAsAtomicUnit=on
  Compare To Constant : simulink/Logic and Bit Operations/Compare To Constant  relop===  const=C_TOS_OFMObjIDInvilad_Val  OutDataTypeStr=boolean
      settings: AttributesFormatString=C_TOS_OFMObjIDInvilad_Val = 0
  For Each : ForEach  DisableCoverage=on
  If : If  IfExpression=u1 ~= 0
  Merge{,1,3..5} (5 alike) : Merge
  TOS_ACC_TargetPre_Confirm_FiltFlag : Outport  ConcatenationDimension=1
  TOS_ACC_TargetPre_FusionTypeFlag_ObserVale : Outport  Port=2  ConcatenationDimension=1
  TOS_ACC_TargetPre_PassedbyTarget_ObserVale : Outport  Port=3  ConcatenationDimension=1
  TOS_ACC_TargetPre_ObjType_ObserVale : Outport  Port=4  ConcatenationDimension=1
  TOS_ACC_DyConfirm_ObserVale : Outport  Port=5  ConcatenationDimension=1
  wires:
  PP_ObjFusType_FC_FR_Confirm/1 -> ACC_Object_PreConfirm/2(PP_ObjFusType_FC_FR_Confirm)
  PP_ObjFusType_FR_Confirm/1 -> ACC_Object_PreConfirm/3(PP_ObjFusType_FR_Confirm)
  Compare To Constant/1 -> If/1
  Object_ID/1 -> [Object_ID], Compare To Constant/1
  If/1 -> ACC_Object_PreConfirmDefault/Action
  If/2 -> ACC_Object_PreConfirm/Action
  PP_ObjFusType_FC_Confirm/1 -> ACC_Object_PreConfirm/4(PP_ObjFusType_FC_Confirm)
  Obj_MovingState/1 -> ACC_Object_PreConfirm/5(Obj_MovingState)
  Obj_Dx/1 -> ACC_Object_PreConfirm/6(Obj_Dx)
  Object_ObstacleProb/1 -> ACC_Object_PreConfirm/7(Object_ObstacleProb)
  Object_DY/1 -> ACC_Object_PreConfirm/8(Object_DY)
  ACC_Target_ID_K1/1 -> ACC_Object_PreConfirm/10(ACC_Target_ID_K1)
  ACC_Target_Dx_K1/1 -> ACC_Object_PreConfirm/11(ACC_Target_Dx_K1)
  [Object_ID] -> ACC_Object_PreConfirm/1(Object_ID)
  Object_ObjType/1 -> ACC_Object_PreConfirm/9(Object_ObjType)
  ACC_Object_PreConfirm/1(TOS_ACC_TargetPre_Confirm_FiltFlag) -> Merge/2
  ACC_Object_PreConfirm/2(TOS_ACC_TargetPre_FusionTypeFlag_ObserVale) -> Merge5/2
  ACC_Object_PreConfirm/3(TOS_ACC_TargetPre_PassedbyTarget_ObserVale) -> Merge1/2
  ACC_Object_PreConfirm/4(TOS_ACC_TargetPre_ObjType_ObserVale) -> Merge3/2
  ACC_Object_PreConfirm/5(TOS_ACC_DyConfirm_ObserVale) -> Merge4/2
  ACC_Object_PreConfirmDefault/1(TOS_ACC_TargetPre_Confirm_FiltFlag) -> Merge/1
  ACC_Object_PreConfirmDefault/2(TOS_ACC_TargetPre_FusionTypeFlag_ObserVale) -> Merge5/1
  ACC_Object_PreConfirmDefault/3(TOS_ACC_TargetPre_PassedbyTarget_ObserVale) -> Merge1/1
  ACC_Object_PreConfirmDefault/4(TOS_ACC_TargetPre_ObjType_ObserVale) -> Merge3/1
  ACC_Object_PreConfirmDefault/5(TOS_ACC_DyConfirm_ObserVale) -> Merge4/1
  Merge/1 -> TOS_ACC_TargetPre_Confirm_FiltFlag/1
  Merge5/1 -> TOS_ACC_TargetPre_FusionTypeFlag_ObserVale/1
  Merge1/1 -> TOS_ACC_TargetPre_PassedbyTarget_ObserVale/1
  Merge3/1 -> TOS_ACC_TargetPre_ObjType_ObserVale/1
  Merge4/1 -> TOS_ACC_DyConfirm_ObserVale/1

== system PubIfDecisionTOS_MDL/TOS_20201112/TOS_2012080320/TOS/ACC/TOS_ACCRightLane/ACC_LeftLane_Target/TOS_ACC_P3 ==
  TOS_ACC_P3_P5_Index : Inport
  Object_ID : Inport  Port=2
  Object_Fus_Type : Inport  Port=3
  object_MovingState : Inport  Port=4
  PP_ObjMovingDirSignalProcessing : Inport  Port=5
  Object_HeadingAngle : Inport  Port=6
  Object_DX : Inport  Port=7
  Object_Type : Inport  Port=8
  Object_ObstacleProb : Inport  Port=9
  Object_DY : Inport  Port=10
  PP_ObjFusType_FC_FR_Confirm : Inport  Port=11
  PP_ObjFusType_FR_Confirm : Inport  Port=12
  PP_ObjFusType_FC_Confirm : Inport  Port=13
  Object_VX : Inport  Port=14
  Object_VY : Inport  Port=15
  VIE_EgoVelocity : Inport  Port=16
  SteerWheelAng : Inport  Port=17
  ACC_TargetP3_ID_K1 : Inport  Port=18
  ACC_TargetP3_ID_K2 : Inport  Port=19
  ACC_TargetP3_MovState_K1 : Inport  Port=20
  ACC_TargetP3_MovState_K2 : Inport  Port=21
  ACC_P3_Targe : Subsystem
  ACC_P3_TargeDefault : Subsystem  TreatAsAtomicUnit=on
  Compare To Constant : simulink/Logic and Bit Operations/Compare To Constant  relop===  const=C_TOS_OFMObjIDInvilad_Val  OutDataTypeStr=boolean
      settings: AttributesFormatString=C_TOS_OFMObjIDInvilad_Val = 0
  Constant1 : Constant  Value=0  OutDataTypeStr=uint8
  If : If  IfExpression=u1 ~= 0
  Merge{,1..5,7..12} (12 alike) : Merge
  Selector17 : Selector  InputPortWidth=2  IndexOptions=Index vector (dialog)  Indices=1  OutputSizes=1
  Switch1 : Switch  Criteria=u2 ~= 0
  TOS_ACC_P3_Index : Outport
  TOS_ACC_FusionType_ObserVale : Outport  Port=2
  TOS_ACC_TrgMovDir_ObserVale : Outport  Port=3
  TOS_ACC_TargetDxConfirm_ObserVale : Outport  Port=4
  TOS_ACC_ObjType_ObserVale : Outport  Port=5
  TOS_ACC_ObstacleProb_ObserVale : Outport  Port=6
  TOS_ACC_TrgMovDirFlag_1_ObserVale : Outport  Port=7
  TOS_ACC_TrgMovDirFlag_2_ObserVale : Outport  Port=8
  TOS_ACC_TrgMovDirFlag_3_ObserVale : Outport  Port=9
  TOS_ACC_TrgMovDirFlag_4_ObserVale : Outport  Port=10
  TOS_ACC_TrgMovDirFlag_5_ObserVale : Outport  Port=11
  TOS_ACC_TrgMovDirFlag_6_ObserVale : Outport  Port=12
  wires:
  ACC_P3_TargeDefault/12(TOS_ACC_TrgMovDirFlag_6_ObserVale) -> Merge8/1
  ACC_P3_TargeDefault/11(TOS_ACC_TrgMovDirFlag_5_ObserVale) -> Merge12/1
  ACC_P3_TargeDefault/10(TOS_ACC_TrgMovDirFlag_4_ObserVale) -> Merge11/1
  ACC_P3_TargeDefault/9(TOS_ACC_TrgMovDirFlag_3_ObserVale) -> Merge10/1
  ACC_P3_TargeDefault/8(TOS_ACC_TrgMovDirFlag_2_ObserVale) -> Merge9/1
  ACC_P3_TargeDefault/7(TOS_ACC_TrgMovDirFlag_1_ObserVale) -> Merge7/1
  ACC_P3_TargeDefault/6(TOS_ACC_ObstacleProb_ObserVale) -> Merge5/1
  ACC_P3_TargeDefault/5(TOS_ACC_ObjType_ObserVale) -> Merge4/1
  ACC_P3_TargeDefault/4(TOS_ACC_TargetDxConfirm_ObserVale) -> Merge3/1
  ACC_P3_TargeDefault/3(TOS_ACC_TrgMovDir_ObserVale) -> Merge2/1
  ACC_P3_TargeDefault/2(TOS_ACC_FusionType_ObserVale) -> Merge1/1
  ACC_P3_TargeDefault/1(ACC_P3_TargeConfirm) -> Merge/1
  Switch1/1 -> TOS_ACC_P3_Index/1
  Selector17/1 -> Compare To Constant/1, [ACC_P3_Index]
  ACC_P3_Targe/11(TOS_ACC_TrgMovDirFlag_5_ObserVale) -> Merge12/2
  ACC_P3_Targe/10(TOS_ACC_TrgMovDirFlag_4_ObserVale) -> Merge11/2
  ACC_P3_Targe/9(TOS_ACC_TrgMovDirFlag_3_ObserVale) -> Merge10/2
  ACC_P3_Targe/8(TOS_ACC_TrgMovDirFlag_2_ObserVale) -> Merge9/2
  Merge12/1 -> TOS_ACC_TrgMovDirFlag_5_ObserVale/1
  Merge11/1 -> TOS_ACC_TrgMovDirFlag_4_ObserVale/1
  Merge10/1 -> TOS_ACC_TrgMovDirFlag_3_ObserVale/1
  Merge9/1 -> TOS_ACC_TrgMovDirFlag_2_ObserVale/1
  Merge8/1 -> TOS_ACC_TrgMovDirFlag_6_ObserVale/1
  ACC_P3_Targe/12(TOS_ACC_TrgMovDirFlag_6_ObserVale) -> Merge8/2
  Object_ID/1 -> ACC_P3_Targe/21(ObjectID)
  ACC_TargetP3_MovState_K2/1 -> ACC_P3_Targe/20(ACC_Target_MovState_K2)
  ACC_TargetP3_MovState_K1/1 -> ACC_P3_Targe/19(ACC_Target_MovState_K1)
  ACC_TargetP3_ID_K2/1 -> ACC_P3_Targe/18(ACC_Target_ID_K2)
  ACC_TargetP3_ID_K1/1 -> ACC_P3_Targe/17(ACC_Target_ID_K1)
  Merge7/1 -> TOS_ACC_TrgMovDirFlag_1_ObserVale/1
  ACC_P3_Targe/7(TOS_ACC_TrgMovDirFlag_1_ObserVale) -> Merge7/2
  SteerWheelAng/1 -> ACC_P3_Targe/16(SteerWheelAng)
  VIE_EgoVelocity/1 -> ACC_P3_Targe/15(VIE_EgoVelocity)
  Object_VX/1 -> ACC_P3_Targe/13(Object_VX)
  Object_VY/1 -> ACC_P3_Targe/14(Object_VY)
  PP_ObjFusType_FR_Confirm/1 -> ACC_P3_Targe/11(PP_ObjFusType_FR_Confirm)
  PP_ObjFusType_FC_FR_Confirm/1 -> ACC_P3_Targe/10(PP_ObjFusType_FC_FR_Confirm)
  PP_ObjFusType_FC_Confirm/1 -> ACC_P3_Targe/12(PP_ObjFusType_FC_Confirm)
  If/2 -> ACC_P3_Targe/Action
  ACC_P3_Targe/6(TOS_ACC_ObstacleProb_ObserVale) -> Merge5/2
  ACC_P3_Targe/5(TOS_ACC_ObjType_ObserVale) -> Merge4/2
  ACC_P3_Targe/4(TOS_ACC_TargetDxConfirm_ObserVale) -> Merge3/2
  ACC_P3_Targe/3(TOS_ACC_TrgMovDir_ObserVale) -> Merge2/2
  ACC_P3_Targe/2(TOS_ACC_FusionType_ObserVale) -> Merge1/2
  ACC_P3_Targe/1(ACC_P3_TargeConfirm) -> Merge/2
  Object_DY/1 -> ACC_P3_Targe/9(Object_DY)
  Object_ObstacleProb/1 -> ACC_P3_Targe/8(Object_ObstacleProb)
  Object_Type/1 -> ACC_P3_Targe/7(Object_Type)
  Object_DX/1 -> ACC_P3_Targe/6(Object_DX)
  Object_HeadingAngle/1 -> ACC_P3_Targe/5(Object_HeadingAngle)
  PP_ObjMovingDirSignalProcessing/1 -> ACC_P3_Targe/4(PP_ObjMovingDirSignalProcessing)
  object_MovingState/1 -> ACC_P3_Targe/3(object_MovingState)
  Object_Fus_Type/1 -> ACC_P3_Targe/2(Object_Fus_Type)
  [ACC_P3_Index] -> ACC_P3_Targe/1(ACC_P3_Index)
  TOS_ACC_P3_P5_Index/1 -> Selector17/1
  Constant1/1 -> Switch1/3
  Merge/1 -> Switch1/2
  [ACC_P3_Index] -> Switch1/1
  Merge5/1 -> TOS_ACC_ObstacleProb_ObserVale/1
  Merge4/1 -> TOS_ACC_ObjType_ObserVale/1
  Merge3/1 -> TOS_ACC_TargetDxConfirm_ObserVale/1
  Merge2/1 -> TOS_ACC_TrgMovDir_ObserVale/1
  Merge1/1 -> TOS_ACC_FusionType_ObserVale/1
  Compare To Constant/1 -> If/1
  If/1 -> ACC_P3_TargeDefault/Action

== system PubIfDecisionTOS_MDL/TOS_20201112/TOS_2012080320/TOS/ACC/TOS_ACCRightLane/ACC_LeftLane_Target/TOS_ACC_P5 ==
  TOS_ACC_P3_P5_Index : Inport
  Object_ID : Inport  Port=2
  Object_Fus_Type : Inport  Port=3
  object_MovingState : Inport  Port=4
  PP_ObjMovingDirSignalProcessing : Inport  Port=5
  Object_HeadingAngle : Inport  Port=6
  Object_DX : Inport  Port=7
  Object_Type : Inport  Port=8
  Object_ObstacleProb : Inport  Port=9
  Object_DY : Inport  Port=10
  PP_ObjFusType_FC_FR_Confirm : Inport  Port=11
  PP_ObjFusType_FR_Confirm : Inport  Port=12
  PP_ObjFusType_FC_Confirm : Inport  Port=13
  Object_VX : Inport  Port=14
  Object_VY : Inport  Port=15
  VIE_EgoVelocity : Inport  Port=16
  SteerWheelAng : Inport  Port=17
  ACC_TargetP5_ID_K1 : Inport  Port=18
  ACC_TargetP5_ID_K2 : Inport  Port=19
  ACC_TargetP5_MovState_K1 : Inport  Port=20
  ACC_TargetP5_MovState_K2 : Inport  Port=21
  ACC_P5_Targe : Subsystem
  ACC_P5_TargeDefault : Subsystem  TreatAsAtomicUnit=on
  Compare To Constant : simulink/Logic and Bit Operations/Compare To Constant  relop===  const=C_TOS_OFMObjIDInvilad_Val  OutDataTypeStr=boolean
      settings: AttributesFormatString=C_TOS_OFMObjIDInvilad_Val = 0
  Constant1 : Constant  Value=0  OutDataTypeStr=uint8
  If : If  IfExpression=u1 ~= 0
  Merge{,1..5,7..12} (12 alike) : Merge
  Selector17 : Selector  InputPortWidth=2  IndexOptions=Index vector (dialog)  Indices=2  OutputSizes=1
  Switch1 : Switch  Criteria=u2 ~= 0
  TOS_ACC_P5_Index : Outport
  TOS_ACC_FusionType_ObserVale : Outport  Port=2
  TOS_ACC_TrgMovDir_ObserVale : Outport  Port=3
  TOS_ACC_TargetDxConfirm_ObserVale : Outport  Port=4
  TOS_ACC_ObjType_ObserVale : Outport  Port=5
  TOS_ACC_ObstacleProb_ObserVale : Outport  Port=6
  TOS_ACC_TrgMovDirFlag_1_ObserVale : Outport  Port=7
  TOS_ACC_TrgMovDirFlag_2_ObserVale : Outport  Port=8
  TOS_ACC_TrgMovDirFlag_3_ObserVale : Outport  Port=9
  TOS_ACC_TrgMovDirFlag_4_ObserVale : Outport  Port=10
  TOS_ACC_TrgMovDirFlag_5_ObserVale : Outport  Port=11
  TOS_ACC_TrgMovDirFlag_6_ObserVale : Outport  Port=12
  wires:
  If/1 -> ACC_P5_TargeDefault/Action
  Compare To Constant/1 -> If/1
  Merge1/1 -> TOS_ACC_FusionType_ObserVale/1
  Merge2/1 -> TOS_ACC_TrgMovDir_ObserVale/1
  Merge3/1 -> TOS_ACC_TargetDxConfirm_ObserVale/1
  Merge4/1 -> TOS_ACC_ObjType_ObserVale/1
  Merge5/1 -> TOS_ACC_ObstacleProb_ObserVale/1
  [ACC_P5_Index] -> Switch1/1
  Merge/1 -> Switch1/2
  Constant1/1 -> Switch1/3
  TOS_ACC_P3_P5_Index/1 -> Selector17/1
  [ACC_P5_Index] -> ACC_P5_Targe/1(ACC_P5_Index)
  Object_Fus_Type/1 -> ACC_P5_Targe/2(Object_Fus_Type)
  object_MovingState/1 -> ACC_P5_Targe/3(object_MovingState)
  PP_ObjMovingDirSignalProcessing/1 -> ACC_P5_Targe/4(PP_ObjMovingDirSignalProcessing)
  Object_HeadingAngle/1 -> ACC_P5_Targe/5(Object_HeadingAngle)
  Object_DX/1 -> ACC_P5_Targe/6(Object_DX)
  Object_Type/1 -> ACC_P5_Targe/7(Object_Type)
  Object_ObstacleProb/1 -> ACC_P5_Targe/8(Object_ObstacleProb)
  Object_DY/1 -> ACC_P5_Targe/9(Object_DY)
  ACC_P5_Targe/1(ACC_P5_TargeConfirm) -> Merge/2
  ACC_P5_Targe/2(TOS_ACC_FusionType_ObserVale) -> Merge1/2
  ACC_P5_Targe/3(TOS_ACC_TrgMovDir_ObserVale) -> Merge2/2
  ACC_P5_Targe/4(TOS_ACC_TargetDxConfirm_ObserVale) -> Merge3/2
  ACC_P5_Targe/5(TOS_ACC_ObjType_ObserVale) -> Merge4/2
  ACC_P5_Targe/6(TOS_ACC_ObstacleProb_ObserVale) -> Merge5/2
  If/2 -> ACC_P5_Targe/Action
  PP_ObjFusType_FC_Confirm/1 -> ACC_P5_Targe/12(PP_ObjFusType_FC_Confirm)
  PP_ObjFusType_FC_FR_Confirm/1 -> ACC_P5_Targe/10(PP_ObjFusType_FC_FR_Confirm)
  PP_ObjFusType_FR_Confirm/1 -> ACC_P5_Targe/11(PP_ObjFusType_FR_Confirm)
  Object_VY/1 -> ACC_P5_Targe/14(Object_VY)
  Object_VX/1 -> ACC_P5_Targe/13(Object_VX)
  VIE_EgoVelocity/1 -> ACC_P5_Targe/15(VIE_EgoVelocity)
  SteerWheelAng/1 -> ACC_P5_Targe/16(SteerWheelAng)
  ACC_P5_Targe/7(TOS_ACC_TrgMovDirFlag_1_ObserVale) -> Merge7/2
  Merge7/1 -> TOS_ACC_TrgMovDirFlag_1_ObserVale/1
  ACC_TargetP5_ID_K1/1 -> ACC_P5_Targe/17(ACC_Target_ID_K1)
  ACC_TargetP5_ID_K2/1 -> ACC_P5_Targe/18(ACC_Target_ID_K2)
  ACC_TargetP5_MovState_K1/1 -> ACC_P5_Targe/19(ACC_Target_MovState_K1)
  ACC_TargetP5_MovState_K2/1 -> ACC_P5_Targe/20(ACC_Target_MovState_K2)
  Object_ID/1 -> ACC_P5_Targe/21(ObjectID)
  ACC_P5_Targe/12(TOS_ACC_TrgMovDirFlag_6_ObserVale) -> Merge8/2
  Merge8/1 -> TOS_ACC_TrgMovDirFlag_6_ObserVale/1
  Merge9/1 -> TOS_ACC_TrgMovDirFlag_2_ObserVale/1
  Merge10/1 -> TOS_ACC_TrgMovDirFlag_3_ObserVale/1
  Merge11/1 -> TOS_ACC_TrgMovDirFlag_4_ObserVale/1
  Merge12/1 -> TOS_ACC_TrgMovDirFlag_5_ObserVale/1
  ACC_P5_Targe/8(TOS_ACC_TrgMovDirFlag_2_ObserVale) -> Merge9/2
  ACC_P5_Targe/9(TOS_ACC_TrgMovDirFlag_3_ObserVale) -> Merge10/2
  ACC_P5_Targe/10(TOS_ACC_TrgMovDirFlag_4_ObserVale) -> Merge11/2
  ACC_P5_Targe/11(TOS_ACC_TrgMovDirFlag_5_ObserVale) -> Merge12/2
  Selector17/1 -> [ACC_P5_Index], Compare To Constant/1
  Switch1/1 -> TOS_ACC_P5_Index/1
  ACC_P5_TargeDefault/1(ACC_P5_TargeConfirm) -> Merge/1
  ACC_P5_TargeDefault/2(TOS_ACC_FusionType_ObserVale) -> Merge1/1
  ACC_P5_TargeDefault/3(TOS_ACC_TrgMovDir_ObserVale) -> Merge2/1
  ACC_P5_TargeDefault/4(TOS_ACC_TargetDxConfirm_ObserVale) -> Merge3/1
  ACC_P5_TargeDefault/5(TOS_ACC_ObjType_ObserVale) -> Merge4/1
  ACC_P5_TargeDefault/6(TOS_ACC_ObstacleProb_ObserVale) -> Merge5/1
  ACC_P5_TargeDefault/7(TOS_ACC_TrgMovDirFlag_1_ObserVale) -> Merge7/1
  ACC_P5_TargeDefault/8(TOS_ACC_TrgMovDirFlag_2_ObserVale) -> Merge9/1
  ACC_P5_TargeDefault/9(TOS_ACC_TrgMovDirFlag_3_ObserVale) -> Merge10/1
  ACC_P5_TargeDefault/10(TOS_ACC_TrgMovDirFlag_4_ObserVale) -> Merge11/1
  ACC_P5_TargeDefault/11(TOS_ACC_TrgMovDirFlag_5_ObserVale) -> Merge12/1
  ACC_P5_TargeDefault/12(TOS_ACC_TrgMovDirFlag_6_ObserVale) -> Merge8/1
